simulink model "attitude_comp_filter"  (R2023a)
settings: configuration reference "configuration_filter" (kept outside this file)
undefined symbols (not defined in the file): dead_reckoning_bool, DiscIntNeverNeededParam, Eul_rad, filt, rot_K_est_OB_B_radDs, sfor_est_B_mDs, sim, x_est
libraries: lib_kinematics x4
settings Model: Creator=FC_dev1  LastModifiedBy=FC_dev1
settings ConfigSetRef: SourceName=configuration_filter  SourceLocation=Base Workspace

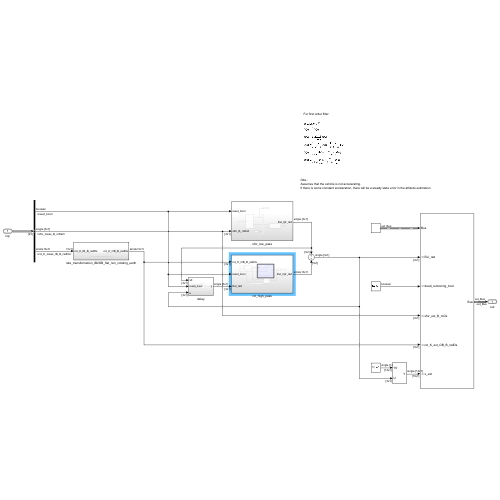
[thumbnail: Simulink's stored preview of the top-level diagram]
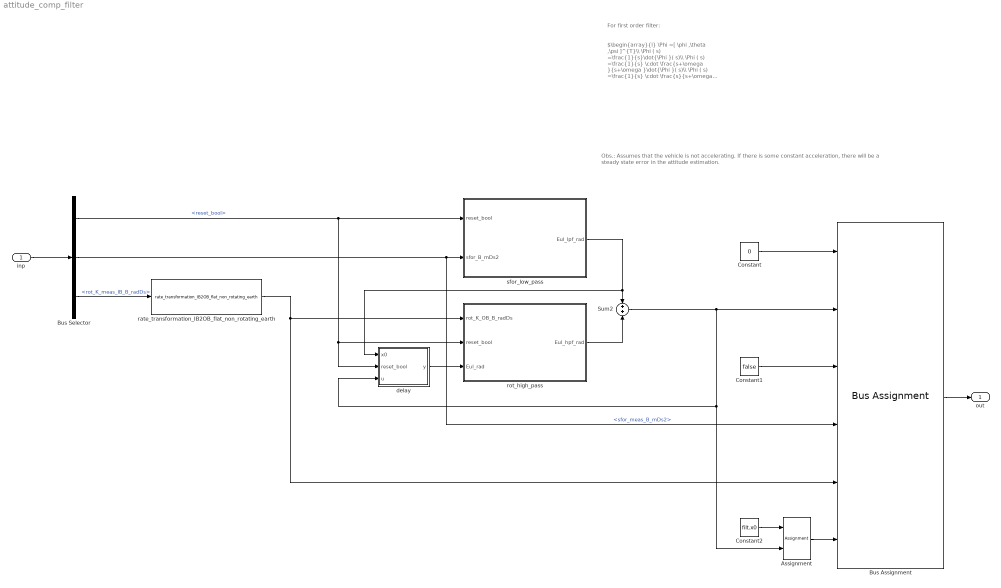
== system attitude_comp_filter ==
  note: Obs.:
      | Assumes that the vehicle is not accelerating.
      | If there is some constant acceleration, there will be a steady state error in the attitude estimation.
  note: For first order filter:
  note: $\begin{array}{l} \Phi =[ \phi ,\theta ,\psi ]^{T}\\ \Phi ( s) =\frac{1}{s}\dot{\Phi }( s)\\ \Phi ( s) =\frac{1}{s} \cdot \frac{s+\omega }{s+\omega }\dot{\Phi }( s)\\ \Phi ( s) =\frac{1}{s} \cdot \frac{s}{s+\omega }\dot{\Phi }( s) +\frac{1}{s} \cdot \frac{\omega }{s+\omega }\dot{\Phi }( s)\\ \Phi ( s) =\frac{1}{s+\omega }\dot{\Phi }( s) +\frac{\omega }{s+\omega } \cdot \frac{1}{s}\dot{\Phi }( s)\\ \Phi ( s) =\frac{1}{s+\omega }\underbrace{\dot{\Phi }( s)}_{gyro} +\frac{\omega }{s+\omega } \cdot \underbrace{\Phi ( s)}_{acc} \end{array}$
  inp : Inport  OutDataTypeStr=Bus: inp_Bus
  Assignment : Assignment  NumberOfDimensions=2  DiagnosticForDimensions=Warning  IndexOptions=Index vector (dialog),Index vector (dialog)  Indices=filt.eul_idx,1  OutputSizes=1,1
  Bus Assignment : BusAssignment  AssignedSignals=Eul_rad,dead_reckoning_bool,sfor_est_B_mDs,rot_K_est_OB_B_radDs,x_est
  Bus Selector : BusSelector  OutputSignals=reset_bool,sfor_meas_B_mDs2,rot_K_meas_IB_B_radDs
  Constant : Constant  Value=0  OutDataTypeStr=Bus: out_Bus
  Constant1 : Constant  Value=false
  Constant2 : Constant  Value=filt.x0  VectorParams1D=off
  Sum2 : Sum
  delay : Subsystem
  rate_transformation_IB2OB_flat_non_rotating_earth : lib_kinematics/rate_transformation_IB2OB_flat_non_rotating_earth  SystemSampleTime=-1  VariantActivationTime=update diagram  Latency=0  AutoFrameSizeCalculation=off
  rot_high_pass : Subsystem
  sfor_low_pass : Subsystem
  out : Outport  OutDataTypeStr=Bus: out_Bus
  wires:
  Bus Selector/2 -> sfor_low_pass/2(sfor_B_mDs2), Bus Assignment/4  "<sfor_meas_B_mDs2>"
  Bus Selector/3 -> rate_transformation_IB2OB_flat_non_rotating_earth/1  "<rot_K_meas_IB_B_radDs>"
  Constant/1 -> Bus Assignment/1
  Bus Assignment/1 -> out/1
  inp/1 -> Bus Selector/1
  rot_high_pass/1(Eul_hpf_rad) -> Sum2/2
  sfor_low_pass/1(Eul_lpf_rad) -> Sum2/1, delay/1(x0)
  Constant1/1 -> Bus Assignment/3
  rate_transformation_IB2OB_flat_non_rotating_earth/1 -> rot_high_pass/1(rot_K_OB_B_radDs), Bus Assignment/5
  Bus Selector/1 -> delay/2(reset_bool), rot_high_pass/2(reset_bool), sfor_low_pass/1(reset_bool)  "<reset_bool>"
  delay/1(y) -> rot_high_pass/3(Eul_rad)
  Constant2/1 -> Assignment/1
  Sum2/1 -> delay/3(u), Assignment/2, Bus Assignment/2
  Assignment/1 -> Bus Assignment/6

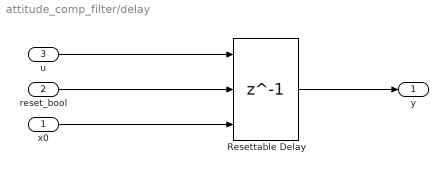
== system attitude_comp_filter/delay ==
  x0 : Inport
  reset_bool : Inport  Port=2
  u : Inport  Port=3
  Resettable Delay : Delay  DelayLength=1  InitialConditionSource=Input port  ExternalReset=Level
      settings: InputPortMap=u0,r5,p4
  y : Outport
  wires:
  reset_bool/1 -> Resettable Delay/2
  u/1 -> Resettable Delay/1
  Resettable Delay/1 -> y/1
  x0/1 -> Resettable Delay/3

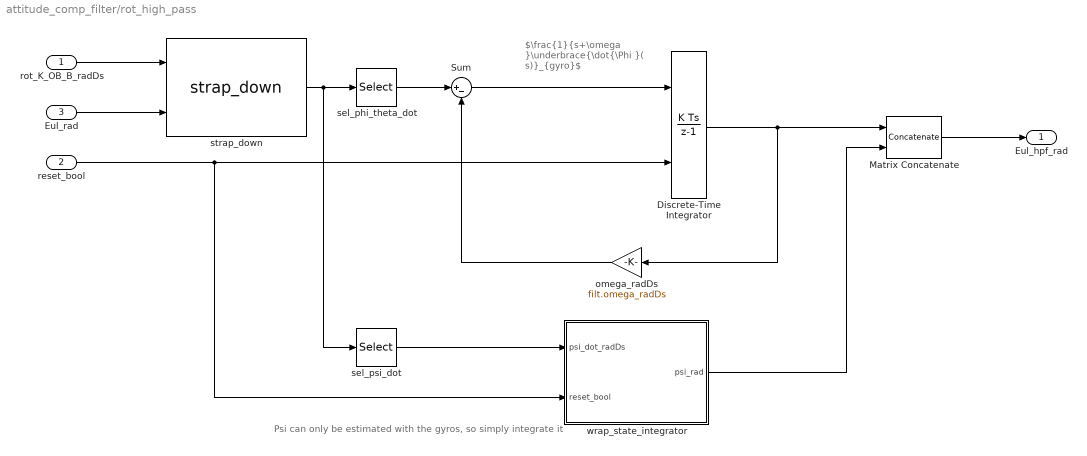
== system attitude_comp_filter/rot_high_pass ==
  note: $\frac{1}{s+\omega }\underbrace{\dot{\Phi }( s)}_{gyro}$
  note: Psi can only be estimated with the gyros, so simply integrate it
  rot_K_OB_B_radDs : Inport
  reset_bool : Inport  Port=2
  Eul_rad : Inport  Port=3
  Discrete-Time Integrator : DiscreteIntegrator  ExternalReset=level  SampleTime=sim.sample_time_s  ICPrevOutput=DiscIntNeverNeededParam  ICPrevScaledInput=DiscIntNeverNeededParam
  Matrix Concatenate : Concatenate  Mode=Multidimensional array
  Sum : Sum  Inputs=|+-
  omega_radDs : Gain  Gain=filt.omega_radDs
  sel_phi_theta_dot : Selector  NumberOfDimensions=2  InputPortWidth=3  IndexOptions=Index vector (dialog),Index vector (dialog)  Indices=[1 2],1  OutputSizes=1,1
  sel_psi_dot : Selector  NumberOfDimensions=2  InputPortWidth=3  IndexOptions=Index vector (dialog),Index vector (dialog)  Indices=3,1  OutputSizes=1,1
  strap_down : lib_kinematics/strap_down  SystemSampleTime=-1  VariantActivationTime=update diagram  Latency=0  AutoFrameSizeCalculation=off
  wrap_state_integrator : Subsystem
  Eul_hpf_rad : Outport
  wires:
  Discrete-Time Integrator/1 -> omega_radDs/1, Matrix Concatenate/1
  Sum/1 -> Discrete-Time Integrator/1
  rot_K_OB_B_radDs/1 -> strap_down/1
  Eul_rad/1 -> strap_down/2
  omega_radDs/1 -> Sum/2
  strap_down/1 -> sel_psi_dot/1, sel_phi_theta_dot/1
  sel_phi_theta_dot/1 -> Sum/1
  Matrix Concatenate/1 -> Eul_hpf_rad/1
  sel_psi_dot/1 -> wrap_state_integrator/1(psi_dot_radDs)
  wrap_state_integrator/1(psi_rad) -> Matrix Concatenate/2
  reset_bool/1 -> wrap_state_integrator/2(reset_bool), Discrete-Time Integrator/2

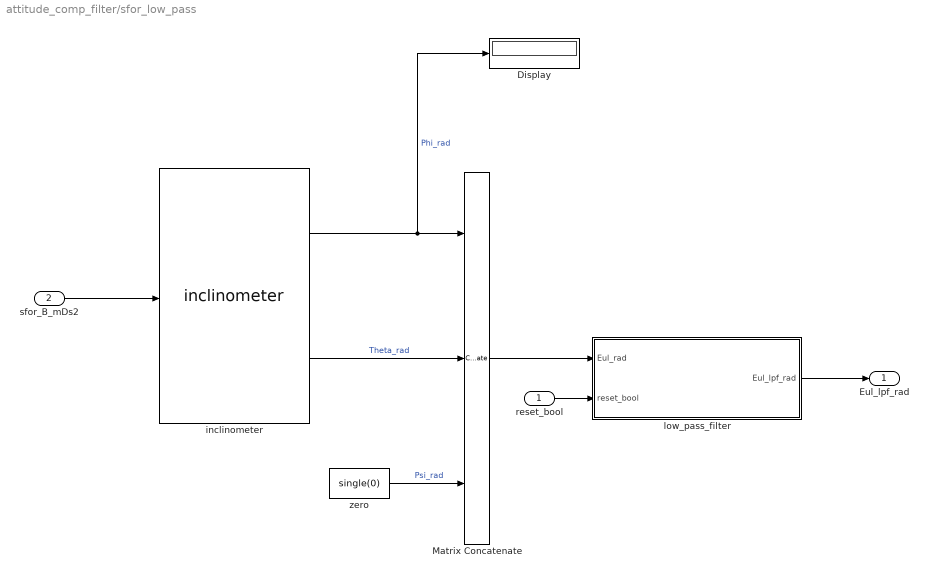
== system attitude_comp_filter/sfor_low_pass ==
  reset_bool : Inport
  sfor_B_mDs2 : Inport  Port=2
  Display : Display
  Matrix Concatenate : Concatenate  NumInputs=3  Mode=Multidimensional array
  inclinometer : lib_kinematics/inclinometer  SystemSampleTime=-1  VariantActivationTime=update diagram  Latency=0  AutoFrameSizeCalculation=off
  low_pass_filter : Subsystem
  zero : Constant  Value=single(0)
  Eul_lpf_rad : Outport
  wires:
  sfor_B_mDs2/1 -> inclinometer/1
  inclinometer/2 -> Matrix Concatenate/2  "Theta_rad"
  zero/1 -> Matrix Concatenate/3  "Psi_rad"
  low_pass_filter/1(Eul_lpf_rad) -> Eul_lpf_rad/1
  Matrix Concatenate/1 -> low_pass_filter/1(Eul_rad)
  inclinometer/1 -> Display/1, Matrix Concatenate/1  "Phi_rad"
  reset_bool/1 -> low_pass_filter/2(reset_bool)

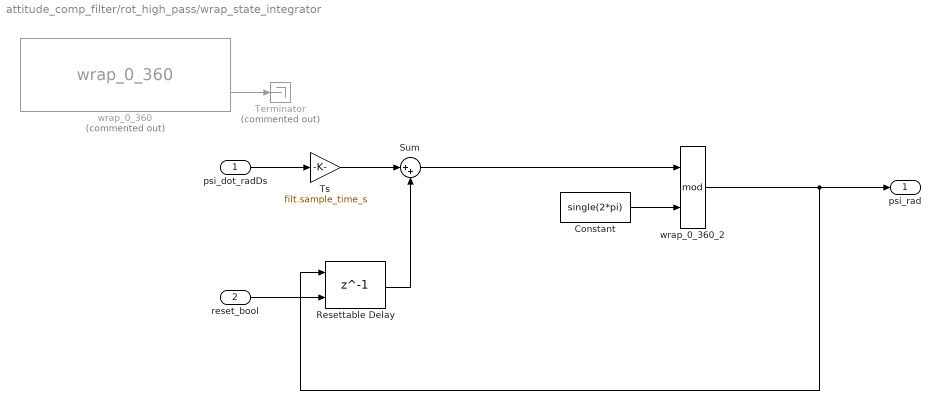
== system attitude_comp_filter/rot_high_pass/wrap_state_integrator ==
  psi_dot_radDs : Inport
  reset_bool : Inport  Port=2
  Constant : Constant  Value=single(2*pi)
  Resettable Delay : Delay  DelayLength=1  InitialCondition=0  ExternalReset=Level
      settings: InputPortMap=u0,r5
  Sum : Sum  Inputs=|++
  Terminator : Terminator  Commented=on
  Ts : Gain  Gain=filt.sample_time_s
  wrap_0_360 : lib_kinematics/wrap_0_360  Commented=on  SystemSampleTime=-1  VariantActivationTime=update diagram  Latency=0  AutoFrameSizeCalculation=off
  wrap_0_360_2 : Math  Operator=mod
  psi_rad : Outport
  wires:
  psi_dot_radDs/1 -> Ts/1
  Ts/1 -> Sum/1
  wrap_0_360/2 -> Terminator/1
  Resettable Delay/1 -> Sum/2
  reset_bool/1 -> Resettable Delay/2
  Sum/1 -> wrap_0_360_2/1
  wrap_0_360_2/1 -> Resettable Delay/1, psi_rad/1
  Constant/1 -> wrap_0_360_2/2

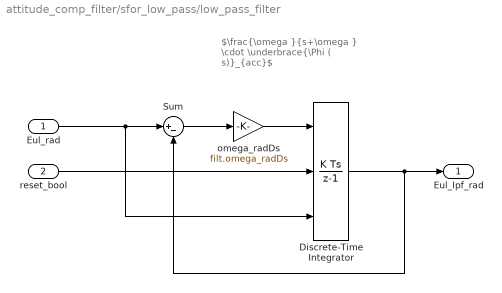
== system attitude_comp_filter/sfor_low_pass/low_pass_filter ==
  note: $\frac{\omega }{s+\omega } \cdot \underbrace{\Phi ( s)}_{acc}$
  Eul_rad : Inport
  reset_bool : Inport  Port=2
  Discrete-Time Integrator : DiscreteIntegrator  ExternalReset=level  InitialConditionSource=external  SampleTime=sim.sample_time_s  ICPrevOutput=DiscIntNeverNeededParam  ICPrevScaledInput=DiscIntNeverNeededParam
  Sum : Sum  Inputs=|+-
  omega_radDs : Gain  Gain=filt.omega_radDs
  Eul_lpf_rad : Outport
  wires:
  omega_radDs/1 -> Discrete-Time Integrator/1
  Discrete-Time Integrator/1 -> Sum/2, Eul_lpf_rad/1
  Sum/1 -> omega_radDs/1
  Eul_rad/1 -> Sum/1, Discrete-Time Integrator/3
  reset_bool/1 -> Discrete-Time Integrator/2
